simulink model "slm5"  (R2018a)
settings: Solver=VariableStepAuto  StartTime=0.0  StopTime=10.0  RelTol=1e-3
values from neighbouring files (symbols this model uses):
  c1 = 116    [setup.m]
  F = 10    [setup.m]
  k1 = 3930    [setup.m]
  k2 = 5720    [setup.m]
settings Model: Creator=Pranav Maddula  LastModifiedBy=Pranav Maddula

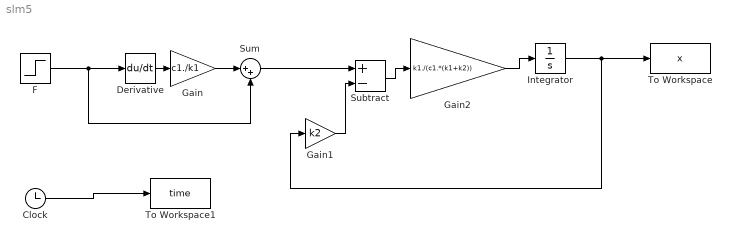
== system slm5 ==
  Clock : Clock
  Derivative : Derivative
  "F " : Step  After=F  SampleTime=0
  Gain : Gain  Gain=c1./k1
  Gain1 : Gain  Gain=k2
  Gain2 : Gain  Gain=k1./(c1.*(k1+k2))
  Integrator : Integrator
  Subtract : Sum  Inputs=+-
  Sum : Sum  Inputs=|++
  To Workspace : ToWorkspace  VariableName=x  SampleTime=-1
  To Workspace1 : ToWorkspace  VariableName=time  SampleTime=-1
  wires:
  Integrator/1 -> Gain1/1, To Workspace/1
  Derivative/1 -> Gain/1
  "F "/1 -> Derivative/1, Sum/2
  Gain/1 -> Sum/1
  Sum/1 -> Subtract/1
  Gain1/1 -> Subtract/2
  Subtract/1 -> Gain2/1
  Gain2/1 -> Integrator/1
  Clock/1 -> To Workspace1/1
